simulink model "test2"  (R2020b)
settings: Solver=VariableStepAuto  StartTime=0.0  StopTime=10.0  RelTol=1e-3
libraries: simulink x1
settings Model: Creator=Luke  LastModifiedBy=Luke

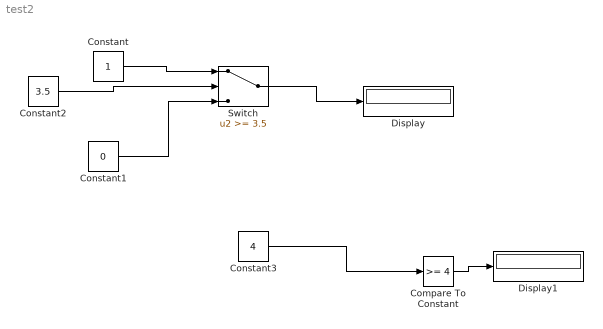
== system test2 ==
  Compare To Constant : simulink/Logic and Bit Operations/Compare To Constant  relop=>=  const=4  OutDataTypeStr=boolean
  Constant : Constant
  Constant1 : Constant  Value=0
  Constant2 : Constant  Value=3.5
  Constant3 : Constant  Value=4
  Display : Display
  Display1 : Display
  Switch : Switch  Threshold=3.5
  wires:
  Constant1/1 -> Switch/3
  Constant/1 -> Switch/1
  Switch/1 -> Display/1
  Constant2/1 -> Switch/2
  Constant3/1 -> Compare To Constant/1
  Compare To Constant/1 -> Display1/1
